simulink model "ForwardKinematicsSim"  (R2020a)
settings: Solver=VariableStepAuto  StartTime=0.0  StopTime=10.0  RelTol=1e-3
settings Model: Creator=Sheldon  LastModifiedBy=Sheldon

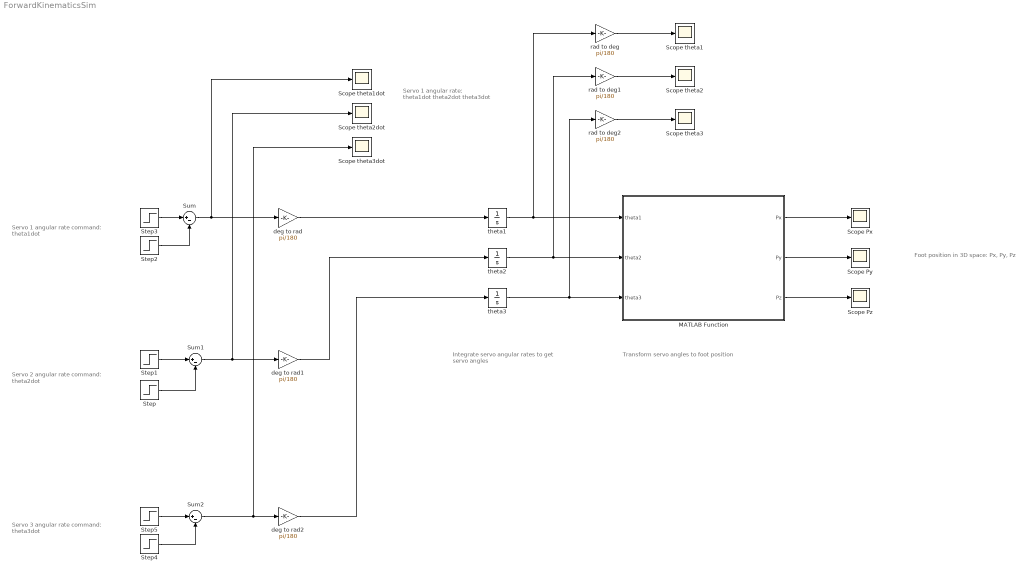
== system ForwardKinematicsSim ==
  note: Servo 1 angular rate
      | command: theta1dot
  note: Servo 2 angular rate
      | command: theta2dot
  note: Servo 3 angular rate
      | command: theta3dot
  note: Servo 1 angular rate:
      |
      | theta1dot
      | theta2dot
      | theta3dot
  note: Integrate servo angular rates to get servo angles
  note: Transform servo angles to foot position
  note: Foot position in 3D space:
      | Px, Py, Pz
  MATLAB Function : MATLAB Function  TreatAsAtomicUnit=on
  Scope Px : Scope
  Scope Py : Scope
  Scope Pz : Scope
  Scope theta1 : Scope
  Scope theta1dot : Scope
  Scope theta2 : Scope
  Scope theta2dot : Scope
  Scope theta3 : Scope
  Scope theta3dot : Scope
  Step{,1,4..5} (4 alike) : Step  SampleTime=0
  Step2 : Step  Time=2  After=10  SampleTime=0
  Step3 : Step  After=10  SampleTime=0
  Sum : Sum  Inputs=|+-
  Sum1 : Sum  Inputs=|+-
  Sum2 : Sum  Inputs=|+-
  deg to rad : Gain  Gain=pi/180
  deg to rad1 : Gain  Gain=pi/180
  deg to rad2 : Gain  Gain=pi/180
  rad to deg : Gain  Gain=pi/180
  rad to deg1 : Gain  Gain=pi/180
  rad to deg2 : Gain  Gain=pi/180
  theta1 : Integrator
  theta2 : Integrator
  theta3 : Integrator
  wires:
  Step3/1 -> Sum/1
  Step2/1 -> Sum/2
  Step1/1 -> Sum1/1
  Step/1 -> Sum1/2
  Step5/1 -> Sum2/1
  Step4/1 -> Sum2/2
  Sum2/1 -> Scope theta3dot/1, deg to rad2/1
  Sum1/1 -> Scope theta2dot/1, deg to rad1/1
  Sum/1 -> Scope theta1dot/1, deg to rad/1
  deg to rad/1 -> theta1/1
  deg to rad1/1 -> theta2/1
  deg to rad2/1 -> theta3/1
  rad to deg/1 -> Scope theta1/1
  rad to deg1/1 -> Scope theta2/1
  rad to deg2/1 -> Scope theta3/1
  theta1/1 -> MATLAB Function/1(theta1), rad to deg/1
  theta2/1 -> MATLAB Function/2(theta2), rad to deg1/1
  theta3/1 -> rad to deg2/1, MATLAB Function/3(theta3)
  MATLAB Function/1(Px) -> Scope Px/1
  MATLAB Function/2(Py) -> Scope Py/1
  MATLAB Function/3(Pz) -> Scope Pz/1

== matlab function ForwardKinematicsSim/MATLAB Function ==
  data: theta1 input; Px output; theta2 input; theta3 input; Py output; Pz output
function [Px,Py,Pz] = fcn(theta1,theta2,theta3)

    % degrees to radians
    d2r = pi/180;

    % Link lengths as defined in Figure 5.3
    L1x = 2;
    L1z = 1;
    L2  = 4;
    L3  = 5;

    % Transformation from servo angles to end effector positions as given in
    % Equation 5.30
    C1  = cos(theta1);
    S1  = sin(theta1);
    C2  = cos(theta2);
    S2  = sin(theta2);
    C23 = cos(theta2 + theta3);
    S23 = sin(theta2 + theta3);

    T03 = [C1*C23, -C1*S23,  S1, C1*(L1x + L3*C23 + L2*C2);...
            S1*C23, -S1*S23, -C1, S1*(L1x + L3*C23 + L2*C2);...
            S23,     C23,   0, L1z + L3*S23 + L2*S2;...
            0,       0,   0, 1];
 
Px = T03(1,4);Py = T03(2,4);Pz = T03(3,4);
